simulink model "motor4"  (R2022b)
settings: Solver=ode15s  StartTime=0.0  StopTime=Tend  RelTol=1e-3
undefined symbols (not defined in the file or in its folder): Bat, ESC, fan, LookUp, motor, Tf, Ts
settings Model: Creator=User  LastModifiedBy=User

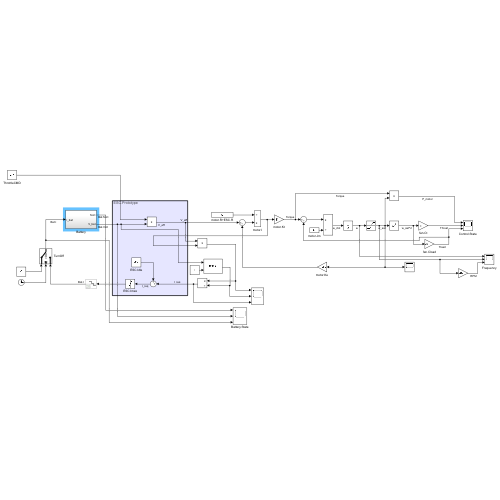
[thumbnail: Simulink's stored preview of the top-level diagram]
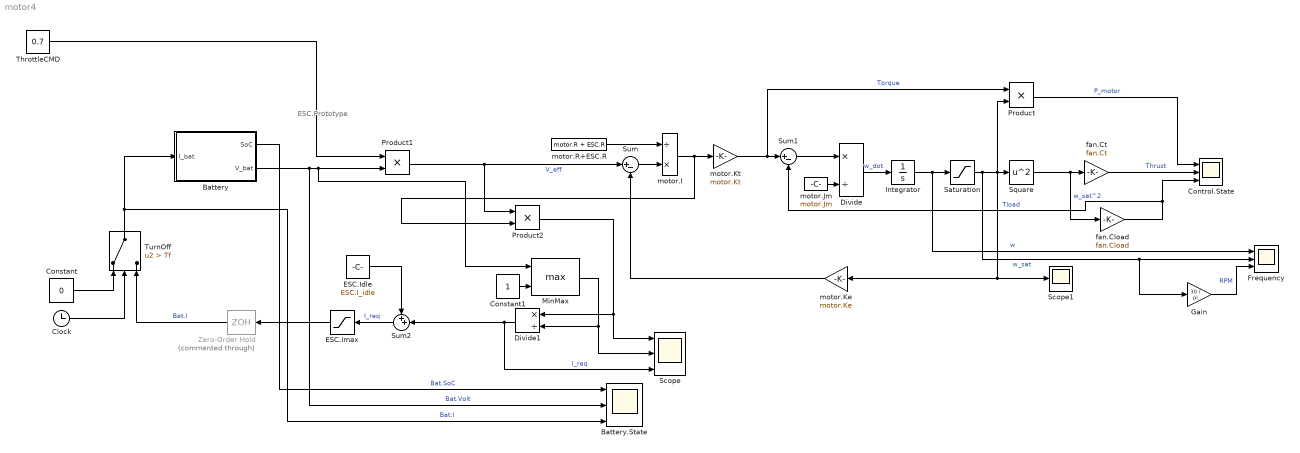
== system motor4 ==
  note: ESC.Prototype
  Battery : Subsystem
  Battery.State : Scope  NumInputPorts=3
  Clock : Clock
  Constant : Constant  Value=0
  Constant1 : Constant
  Control.State : Scope  NumInputPorts=3
  Divide : Product  Inputs=*/
  Divide1 : Product  Inputs=*/
  ESC.Idle : Constant  Value=ESC.I_idle
  ESC.Imax : Saturate  UpperLimit=ESC.Imax
  Frequency : Scope  NumInputPorts=3
  Gain : Gain  Gain=30 / pi
  Integrator : Integrator
  MinMax : MinMax  Function=max  Inputs=2
  Product : Product
  Product1 : Product
  Product2 : Product
  Saturation : Saturate  UpperLimit=motor.maxFreq  LowerLimit=0
  Scope : Scope  NumInputPorts=3
  Scope1 : Scope
  Square : Math  Operator=square
  Sum : Sum  Inputs=|+-
  Sum1 : Sum  Inputs=|+-
  Sum2 : Sum  Inputs=++|
  ThrottleCMD : Constant  Value=0.7
  TurnOff : Switch  Criteria=u2 > Threshold  Threshold=Tf  SaturateOnIntegerOverflow=off  InputSameDT=off
  Zero-Order Hold : ZeroOrderHold  Commented=through  SampleTime=Ts
  fan.Cload : Gain  Gain=fan.Cload
  fan.Ct : Gain  Gain=fan.Ct
  motor.I : Product  Inputs=/*
  motor.Jm : Constant  Value=motor.Jm
  motor.Ke : Gain  Gain=motor.Ke
  motor.Kt : Gain  Gain=motor.Kt
  motor.R+ESC.R : Constant  Value=motor.R + ESC.R
  wires:
  motor.Kt/1 -> Sum1/1, Product/1  "Torque"
  motor.Jm/1 -> Divide/2
  Divide/1 -> Integrator/1  "w_dot"
  Integrator/1 -> Frequency/1, Saturation/1  "w"
  Saturation/1 -> Gain/1, Frequency/2, Product/2, Scope1/1, motor.Ke/1, Square/1  "w_sat"
  Square/1 -> fan.Cload/1, fan.Ct/1  "w_sat^2"
  fan.Ct/1 -> Control.State/2  "Thrust"
  fan.Cload/1 -> Control.State/3, Sum1/2  "Tload"
  motor.Ke/1 -> Sum/2
  Sum/1 -> motor.I/2
  motor.R+ESC.R/1 -> motor.I/1
  motor.I/1 -> Product2/2, motor.Kt/1
  Sum1/1 -> Divide/1
  Product/1 -> Control.State/1  "P_motor"
  Battery/1(SoC) -> Battery.State/1  "Bat.SoC"
  Sum2/1 -> ESC.Imax/1  "I_req"
  Gain/1 -> Frequency/3  "RPM"
  Battery/2(V_bat) -> Battery.State/2, MinMax/1, Product1/2  "Bat.Volt"
  Divide1/1 -> Scope/3, Sum2/2  "I_req"
  ESC.Idle/1 -> Sum2/1
  ESC.Imax/1 -> Zero-Order Hold/1
  TurnOff/1 -> Battery/1(I_bat), Battery.State/3  "Bat.I"
  Zero-Order Hold/1 -> TurnOff/3  "Bat.I"
  Clock/1 -> TurnOff/2
  ThrottleCMD/1 -> Product1/1
  Constant/1 -> TurnOff/1
  Product1/1 -> Product2/1, Sum/1  "V_eff"
  Constant1/1 -> MinMax/2
  Product2/1 -> Scope/1, Divide1/1
  MinMax/1 -> Scope/2, Divide1/2

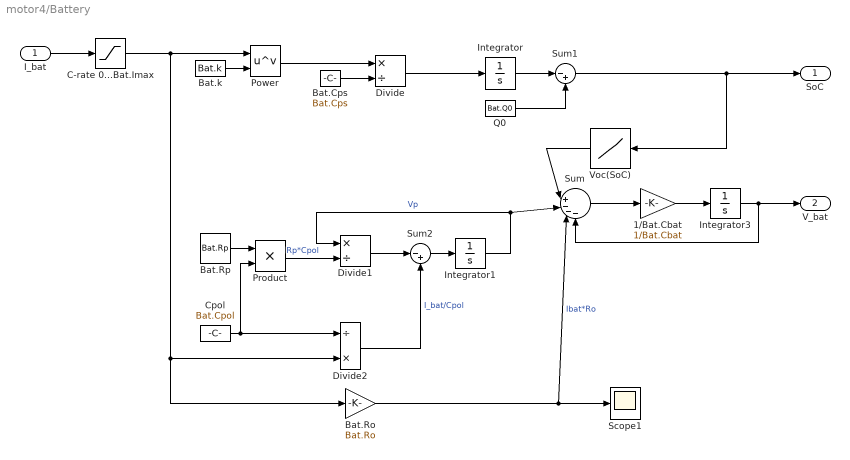
== system motor4/Battery ==
  I_bat : Inport
  1/Bat.Cbat : Gain  Gain=1/Bat.Cbat
  Bat.Cps : Constant  Value=Bat.Cps
  Bat.Ro : Gain  Gain=Bat.Ro
  Bat.Rp : Constant  Value=Bat.Rp
  Bat.k : Constant  Value=Bat.k
  C-rate 0...Bat.Imax : Saturate  UpperLimit=Bat.Imax  LowerLimit=0
  Cpol : Constant  Value=Bat.Cpol
  Divide : Product  Inputs=*/
  Divide1 : Product  Inputs=*/
  Divide2 : Product  Inputs=/*
  Integrator : Integrator
  Integrator1 : Integrator
  Integrator3 : Integrator  InitialCondition=Bat.Vcell*Bat.ncell
  Power : Math  Operator=pow
  Product : Product
  Q0 : Constant  Value=Bat.Q0
  Scope1 : Scope
  Sum : Sum  Inputs=||+---
  Sum1 : Sum  Inputs=|-+
  Sum2 : Sum  Inputs=|-+
  Voc(SoC) : Lookup_n-D  NumberOfTableDimensions=1  BreakpointsForDimension1=LookUp.SoC  Table=LookUp.Volts  InternalRulePriority=Speed  RndMeth=Simplest
  SoC : Outport
  V_bat : Outport  Port=2
  wires:
  Integrator1/1 -> Divide1/1, Sum/2  "Vp"
  Sum2/1 -> Integrator1/1
  Product/1 -> Divide1/2  "Rp*Cpol"
  Q0/1 -> Sum1/2
  Cpol/1 -> Divide2/1, Product/2
  Bat.Rp/1 -> Product/1
  Power/1 -> Divide/1
  Bat.Cps/1 -> Divide/2
  Bat.k/1 -> Power/2
  Sum/1 -> 1/Bat.Cbat/1
  I_bat/1 -> C-rate 0...Bat.Imax/1
  Integrator/1 -> Sum1/1
  Sum1/1 -> Voc(SoC)/1, SoC/1
  Divide1/1 -> Sum2/1
  Divide2/1 -> Sum2/2  "I_bat/Cpol"
  Bat.Ro/1 -> Sum/3, Scope1/1  "Ibat*Ro"
  Divide/1 -> Integrator/1
  C-rate 0...Bat.Imax/1 -> Bat.Ro/1, Divide2/2, Power/1
  Integrator3/1 -> V_bat/1, Sum/4
  1/Bat.Cbat/1 -> Integrator3/1
  Voc(SoC)/1 -> Sum/1
